simulink subsystem "DAC"  (R2024b)
settings: Solver=VariableStepAuto  StartTime=0.0  StopTime=10.0  RelTol=1e-3
values from neighbouring files (symbols this model uses):
  Ts = 1e-3    (= 0.001)    [Plant_EstimTrialUpdateLAB17_04_25.m]
settings Model: Creator=Riccardo Grosso  LastModifiedBy=Riccardo Grosso

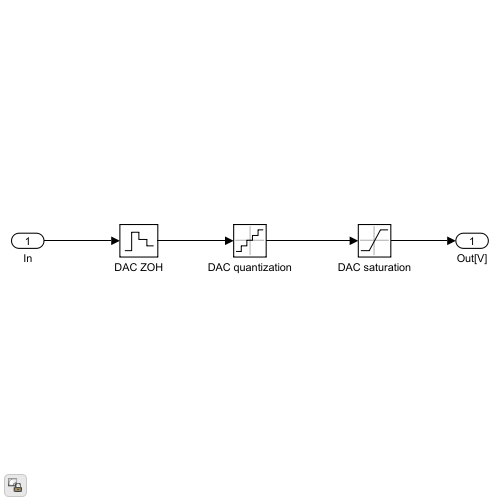
[thumbnail: Simulink's stored preview of the top-level diagram]
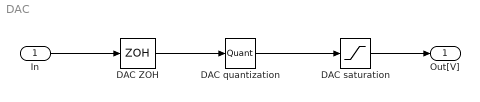
== system DAC ==
  In : Inport
  DAC ZOH : ZeroOrderHold  SampleTime=Ts
  DAC quantization : Quantizer  QuantizationInterval=20/(pow2(16)-1)
  DAC saturation : Saturate  UpperLimit=10  LowerLimit=-10
  Out[V] : Outport  Unit=V
  wires:
  DAC quantization/1 -> DAC saturation/1
  DAC ZOH/1 -> DAC quantization/1
  In/1 -> DAC ZOH/1
  DAC saturation/1 -> Out[V]/1
